simulink model "F16_2023a"  (R2025b)
settings: Solver=VariableStepAuto  StartTime=0.0  StopTime=inf  RelTol=1e-3
values from neighbouring files (symbols this model uses):
  Param = load_F16_params()    [F16AeroFM.m]    (also in runF16.m)
libraries: aerolibasang x3, aerolibfltsims x2, aerolibobsolete x1, aerolibatmos2 x1, sl3dlib x1
settings Model: Creator=sherpa  LastModifiedBy=leonardo
settings SolverCC: AlgebraicLoopSolver=TrustRegion
settings DebuggingCC: UnconnectedInputMsg=warning  UnconnectedOutputMsg=warning  UnconnectedLineMsg=warning
settings ModelReferenceCC: EnableRefExpFcnMdlSchedulingChecks=on
settings RTWCC: GPUComputeCapability=3.5  DLArmComputeVersion=19.05

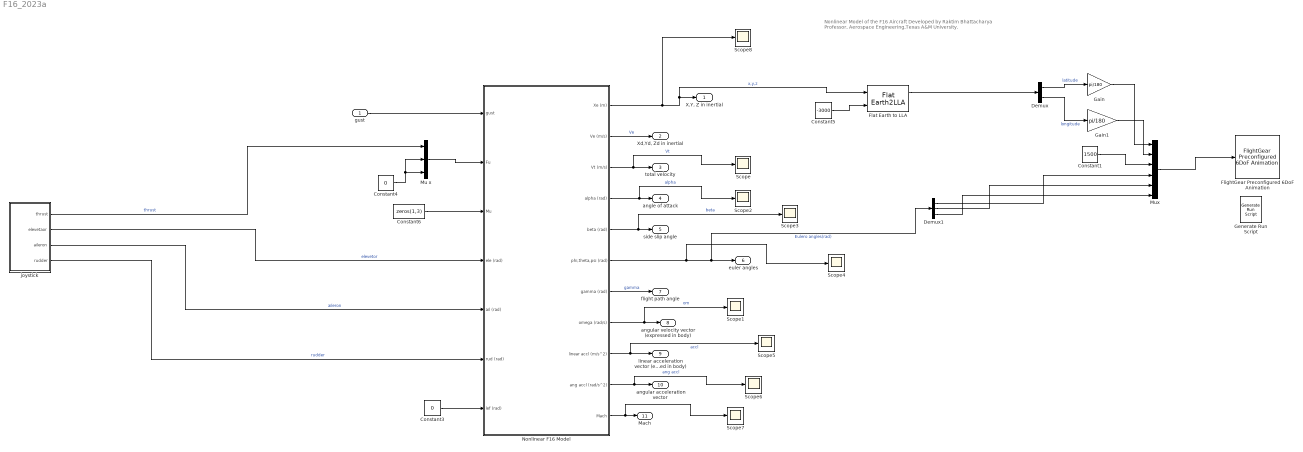
== system F16_2023a ==
  note: Nonlinear Model of the F16 Aircraft
      |
      | Developed by
      |
      | Raktim Bhattacharya
      | Professor,
      | Aerospace Engineering,Texas A&M University.
  gust : Inport
  Constant1 : Constant  Value=1500
  Constant3 : Constant  Value=0
  Constant4 : Constant  Value=0
  Constant5 : Constant  Value=-3000
  Constant6 : Constant  Value=zeros(1,3)
  Demux : Demux  Outputs=2
  Demux1 : Demux  Outputs=3
  Flat Earth to LLA : FlatEarth2LLA  LL0=[0 0]
  FlightGear Preconfigured 6DoF Animation : aerolibfltsims/FlightGear Preconfigured 6DoF Animation  xFlightGearVersion=v2019.1  DestinationIpAddress=127.0.0.1  DestinationPort=5502  SampleTime=1/30  packetVersion=24
  Gain : Gain  Gain=pi/180
  Gain1 : Gain  Gain=pi/180
  Generate Run Script : aerolibfltsims/Generate Run Script  Architecture=Linux  dataFlow=Send  GeometryModelName=c172p  AirportId=LIME  RunwayId=28  InitialAltitude=15000  InitialHeading=0  OffsetDistance=4.72  OffsetAzimuth=0  InstallScenery=off  DisableShaders=on  OriginAddress=127.0.0.1  DestinationPort=5502  OriginPort=5505  LocalAddress=127.0.0.1  OutputFileName=runfg.bat  FlightGearBaseDirectory=/usr/share/games/flightgear
  Mu x : Mux  Inputs=3
  Mux : Mux  Inputs=6
  Nonlinear F16 Model : Subsystem
  Scope{,1..8} (9 alike) : Scope
      Scope settings: ActiveDisplayYMinimum=-2227.5402486379644  ActiveDisplayYMaximum=2188.5768238395149
      Scope1 settings: ActiveDisplayYMinimum=-6.8377151322792935  ActiveDisplayYMaximum=6.6990721082944527
      Scope2 settings: ActiveDisplayYMinimum=-0.59864049768432848  ActiveDisplayYMaximum=0.52158775907311861  DataLoggingVariableName=ScopeData9
      Scope3 settings: ActiveDisplayYMinimum=-1  ActiveDisplayYMaximum=1  DataLoggingVariableName=ScopeData10
      Scope4 settings: ActiveDisplayYMinimum=-11.019979808038256  ActiveDisplayYMaximum=11.25037786436754  DataLoggingVariableName=ScopeData11
      Scope5 settings: DataLoggingVariableName=ScopeData12
      Scope6 settings: ActiveDisplayYMinimum=-1  ActiveDisplayYMaximum=1  DataLoggingVariableName=ScopeData13
      Scope7 settings: ActiveDisplayYMinimum=-1  ActiveDisplayYMaximum=1  DataLoggingVariableName=ScopeData14
      Scope8 settings: ActiveDisplayYMinimum=-126537.06226625846  ActiveDisplayYMaximum=56078.717128878794  DataLoggingVariableName=ScopeData15
  joystick : Subsystem
  "X,Y, Z in inertial" : Outport
  "Xd,Yd, Zd in inertial" : Outport  Port=2
  total velocity : Outport  Port=3
  angle of attack : Outport  Port=4
  side slip angle : Outport  Port=5
  euler angles : Outport  Port=6
  flight path angle : Outport  Port=7
  angular velocity vector (expressed in body) : Outport  Port=8
  linear acceleration vector (expressed in body) : Outport  Port=9
  angular acceleration vector : Outport  Port=10
  Mach : Outport  Port=11
  wires:
  Nonlinear F16 Model/3(Vt (m/s)) -> Scope/1, total velocity/1  "Vt"
  Nonlinear F16 Model/4(alpha (rad)) -> Scope2/1, angle of attack/1  "alpha"
  Nonlinear F16 Model/5(beta (rad)) -> Scope3/1, side slip angle/1  "beta"
  Nonlinear F16 Model/7(gamma (rad)) -> flight path angle/1  "gamma"
  Nonlinear F16 Model/8(omega (rad/s)) -> Scope1/1, angular velocity vector (expressed in body)/1  "om"
  Nonlinear F16 Model/9(linear accl (m/s^2)) -> Scope5/1, linear acceleration vector (expressed in body)/1  "accl"
  Nonlinear F16 Model/2(Ve (m/s)) -> "Xd,Yd, Zd in inertial"/1  "Ve"
  Nonlinear F16 Model/10(ang accl (rad/s^2)) -> Scope6/1, angular acceleration vector/1  "ang accl"
  Nonlinear F16 Model/11(Mach) -> Scope7/1, Mach/1
  Constant3/1 -> Nonlinear F16 Model/7(lef (rad))
  Nonlinear F16 Model/6(phi,theta,psi (rad)) -> Scope4/1, Demux1/1, euler angles/1  "Eulero angles(rad)"
  Nonlinear F16 Model/1(Xe (m)) -> Scope8/1, Flat Earth to LLA/1, "X,Y, Z in inertial"/1  "x,y,z"
  Constant4/1 -> Mu x/2, Mu x/3
  Mu x/1 -> Nonlinear F16 Model/2(Fu)
  Flat Earth to LLA/1 -> Demux/1
  Constant5/1 -> Flat Earth to LLA/2
  Constant6/1 -> Nonlinear F16 Model/3(Mu)
  Demux/1 -> Gain/1  "latitude"
  Demux/2 -> Gain1/1  "longitude"
  Mux/1 -> FlightGear Preconfigured 6DoF Animation/1
  Demux1/1 -> Mux/4
  Demux1/2 -> Mux/5
  Constant1/1 -> Mux/3
  gust/1 -> Nonlinear F16 Model/1(gust)
  joystick/1(thrust) -> Mu x/1  "thrust"
  joystick/2(elevetaor) -> Nonlinear F16 Model/4(ele (rad))  "elevetor"
  joystick/3(aileron) -> Nonlinear F16 Model/5(ail (rad))  "aileron"
  joystick/4(rudder) -> Nonlinear F16 Model/6(rud (rad))  "rudder"
  Demux1/3 -> Mux/6
  Gain/1 -> Mux/1
  Gain1/1 -> Mux/2

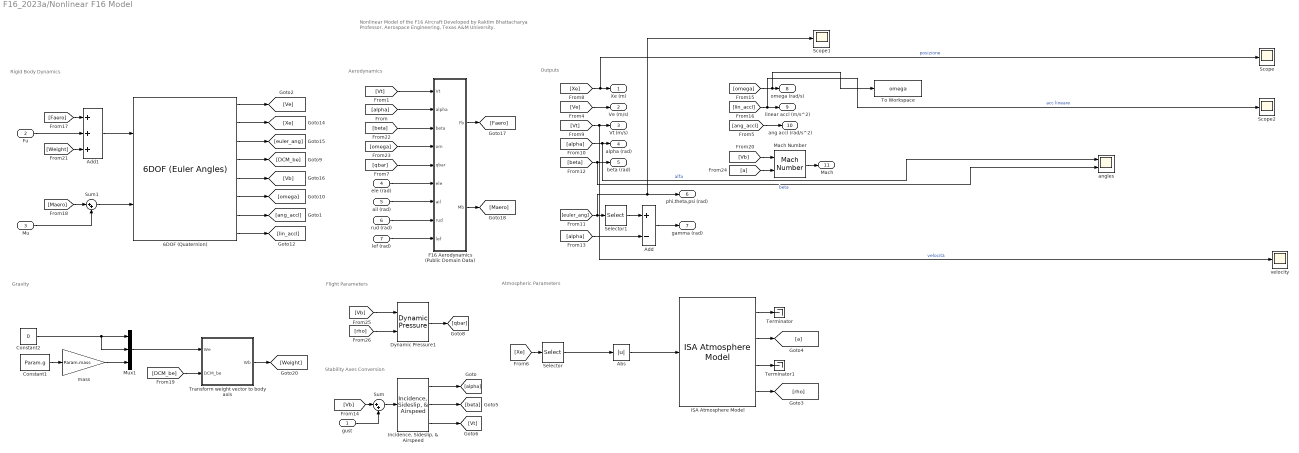
== system F16_2023a/Nonlinear F16 Model ==
  note: Gravity
  note: Nonlinear Model of the F16 Aircraft
      |
      | Developed by Raktim Bhattacharya
      | Professor, Aerospace Engineering,
      | Texas A&M University.
  note: Aerodynamics
  note: Outputs
  note: Rigid Body Dynamics
  note: Stability Axes Conversion
  note: Atmospheric Parameters
  note: Flight Parameters
  gust : Inport  PortDimensions=3
  Fu : Inport  Port=2  PortDimensions=3
  Mu : Inport  Port=3  PortDimensions=3
  ele (rad) : Inport  Port=4
  ail (rad) : Inport  Port=5
  rud (rad) : Inport  Port=6
  lef (rad) : Inport  Port=7
  6DOF (Quaternion) : aerolibobsolete/6DOF (Euler Angles)  units=Metric (MKS)  mtype=Fixed  rep=Euler Angles  xme_0=IC.inertial_position  Vm_0=IC.body_velocity  eul_0=IC.euler_angles  pm_0=IC.omega  mass_0=Param.mass  mass_e=0.5  mass_f=2.0  inertia=Param.moi  inertia_e=eye(3)  inertia_f=2*eye(3)  k_quat=1.0  vre_flag=on  abi_flag=off  aMode=0  xme_statename={'Xe', 'Ye', 'Ze'}  Vm_statename={'U', 'v', 'w'}  eul_statename=''  quat_statename={'qr', 'qi', 'qj', 'qk'}  pm_statename={'p', 'q', 'r'}  mass_statename=''
  Abs : Abs  SaturateOnIntegerOverflow=off
  Add : Sum  Inputs=+-
  Add1 : Sum  Inputs=+++
  Constant1 : Constant  Value=Param.g
  Constant2 : Constant  Value=0
  Dynamic Pressure1 : aerolibasang/Dynamic Pressure
  F16 Aerodynamics (Public Domain Data) : Subsystem
  ISA Atmosphere Model : aerolibatmos2/ISA Atmosphere Model  useExtended=off  action=None  custom=off  viscosityOut=off  g=9.80665  gamma=1.4  R=287.0531  L=0.0065  h_trop=11000  h_strat=20000  rho0=1.225  P0=101325  T0=288.15  h0=0  S=110.4  Tref=273.15  muref=1.716e-5
  "Incidence, Sideslip, & Airspeed" : aerolibasang/Incidence, Sideslip, & Airspeed
  Mach Number : aerolibasang/Mach Number
  Mux1 : Mux  Inputs=3
  Scope : Scope
      settings: ActiveDisplayYMinimum=-9160.141053235342  ActiveDisplayYMaximum=5347.118129523169  DataLoggingVariableName=ScopeData2
  Scope1 : Scope
      settings: ActiveDisplayYMinimum=-2.5924276815871528  ActiveDisplayYMaximum=1.1099100940481796  DataLoggingVariableName=ScopeData3
  Scope2 : Scope
      settings: ActiveDisplayYMinimum=-38.16136847895087  ActiveDisplayYMaximum=61.768795303374354  DataLoggingVariableName=ScopeData5
  Selector : Selector  InputPortWidth=3  IndexOptions=Index vector (dialog)  Indices=3  OutputSizes=1
  Selector1 : Selector  InputPortWidth=3  IndexOptions=Index vector (dialog)  Indices=2  OutputSizes=1
  Sum : Sum  Inputs=|++
  Sum1 : Sum  Inputs=|++
  Terminator : Terminator
  Terminator1 : Terminator
  To Workspace : ToWorkspace  VariableName=omega  SaveFormat=Timeseries  SampleTime=-1
  Transform weight vector to body axis : MATLAB Function  TreatAsAtomicUnit=on
  angles : Scope  NumInputPorts=2
      settings: ActiveDisplayYMinimum=-0.37545003667394233  ActiveDisplayYMaximum=0.11642688367935129  DataLoggingVariableName=ScopeData4
  mass : Gain  Gain=Param.mass
  velocity : Scope
      settings: ActiveDisplayYMinimum=59.795753806398508  ActiveDisplayYMaximum=111.44827585460112  DataLoggingVariableName=ScopeData6
  Xe (m) : Outport
  Ve (m/s) : Outport  Port=2
  Vt (m/s) : Outport  Port=3
  alpha (rad) : Outport  Port=4
  beta (rad) : Outport  Port=5
  phi,theta,psi (rad) : Outport  Port=6
  gamma (rad) : Outport  Port=7
  omega (rad/s) : Outport  Port=8
  linear accl (m/s^2) : Outport  Port=9
  ang accl (rad/s^2) : Outport  Port=10
  Mach : Outport  Port=11
  wires:
  [Xe] -> Selector/1
  [beta] -> angles/2, beta (rad)/1  "beta"
  "Incidence, Sideslip, & Airspeed"/3 -> [Vt]
  ISA Atmosphere Model/3 -> Terminator1/1
  ISA Atmosphere Model/1 -> Terminator/1
  ISA Atmosphere Model/4 -> [rho]
  [lin_accl] -> Scope2/1, linear accl (m/s^2)/1  "acc lineare"
  [alpha] -> angles/1, alpha (rad)/1  "alfa"
  ISA Atmosphere Model/2 -> [a]
  Add/1 -> gamma (rad)/1
  [Vt] -> velocity/1, Vt (m/s)/1  "velocità"
  "Incidence, Sideslip, & Airspeed"/2 -> [beta]
  Selector1/1 -> Add/1
  "Incidence, Sideslip, & Airspeed"/1 -> [alpha]
  Selector/1 -> Abs/1
  [alpha] -> Add/2
  [euler_ang] -> Scope1/1, phi,theta,psi (rad)/1, Selector1/1
  [omega] -> To Workspace/1, omega (rad/s)/1
  [Xe] -> Scope/1, Xe (m)/1  "posizione"
  Constant1/1 -> mass/1
  mass/1 -> Mux1/3
  Mux1/1 -> Transform weight vector to body axis/1(We)
  Transform weight vector to body axis/1(Wb) -> [Weight]
  [DCM_be] -> Transform weight vector to body axis/2(DCM_be)
  Constant2/1 -> Mux1/2, Mux1/1
  [Faero] -> Add1/1
  Fu/1 -> Add1/2
  [Weight] -> Add1/3
  Add1/1 -> 6DOF (Quaternion)/1
  [Vb] -> Sum/1
  Sum/1 -> "Incidence, Sideslip, & Airspeed"/1
  gust/1 -> Sum/2
  [Maero] -> Sum1/1
  Mu/1 -> Sum1/2
  6DOF (Quaternion)/1 -> [Ve]
  6DOF (Quaternion)/2 -> [Xe]
  6DOF (Quaternion)/3 -> [euler_ang]
  6DOF (Quaternion)/4 -> [DCM_be]
  6DOF (Quaternion)/5 -> [Vb]
  6DOF (Quaternion)/6 -> [omega]
  6DOF (Quaternion)/7 -> [ang_accl]
  6DOF (Quaternion)/8 -> [lin_accl]
  [Ve] -> Ve (m/s)/1
  [ang_accl] -> ang accl (rad/s^2)/1
  [Vb] -> Mach Number/1
  [a] -> Mach Number/2
  Mach Number/1 -> Mach/1
  F16 Aerodynamics (Public Domain Data)/1(Fb) -> [Faero]
  Sum1/1 -> 6DOF (Quaternion)/2
  F16 Aerodynamics (Public Domain Data)/2(Mb) -> [Maero]
  [Vt] -> F16 Aerodynamics (Public Domain Data)/1(Vt)
  [alpha] -> F16 Aerodynamics (Public Domain Data)/2(alpha)
  [beta] -> F16 Aerodynamics (Public Domain Data)/3(beta)
  [omega] -> F16 Aerodynamics (Public Domain Data)/4(om)
  [qbar] -> F16 Aerodynamics (Public Domain Data)/5(qbar)
  ele (rad)/1 -> F16 Aerodynamics (Public Domain Data)/6(ele)
  ail (rad)/1 -> F16 Aerodynamics (Public Domain Data)/7(ail)
  rud (rad)/1 -> F16 Aerodynamics (Public Domain Data)/8(rud)
  lef (rad)/1 -> F16 Aerodynamics (Public Domain Data)/9(lef)
  Abs/1 -> ISA Atmosphere Model/1
  Dynamic Pressure1/1 -> [qbar]
  [Vb] -> Dynamic Pressure1/1
  [rho] -> Dynamic Pressure1/2

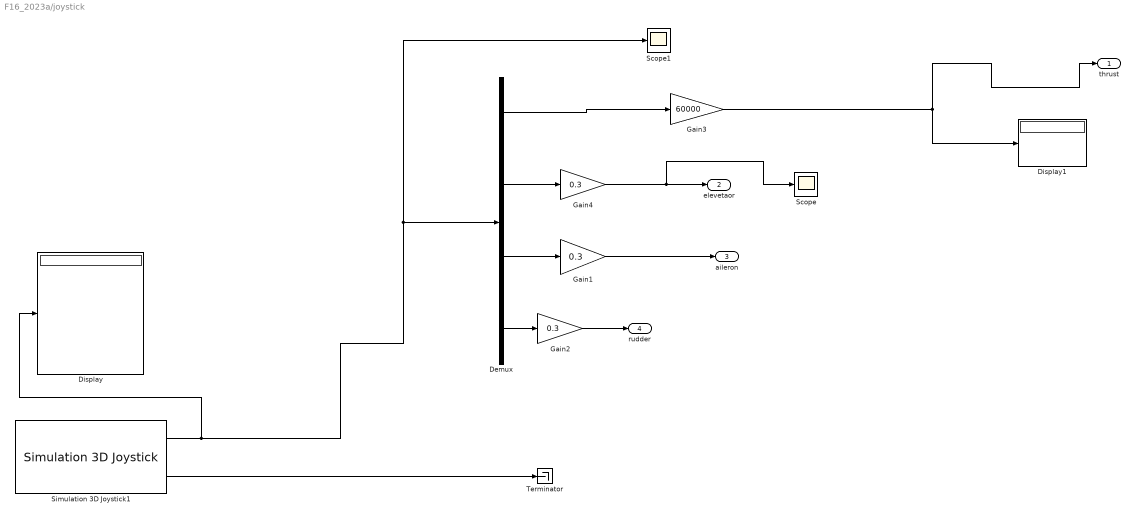
== system F16_2023a/joystick ==
  Demux : Demux
  Display : Display
  Display1 : Display
  Gain1 : Gain  Gain=0.3
  Gain2 : Gain  Gain=0.3
  Gain3 : Gain  Gain=60000
  Gain4 : Gain  Gain=0.3
  Scope : Scope
      settings: ActiveDisplayYMinimum=-0.18749999999999997  ActiveDisplayYMaximum=0.18749999999999997  DataLoggingVariableName=ScopeData7
  Scope1 : Scope
      settings: ActiveDisplayYMinimum=-12.345890787364121  ActiveDisplayYMaximum=10.806609212635932  DataLoggingVariableName=ScopeData8
  Simulation 3D Joystick1 : sl3dlib/Simulation 3D/Hardware Interface/Simulation 3D Joystick  joyid=1  adjustports=on  forcefeed=off
  Terminator : Terminator
  thrust : Outport
  elevetaor : Outport  Port=2
  aileron : Outport  Port=3
  rudder : Outport  Port=4
  wires:
  Gain4/1 -> Scope/1, elevetaor/1
  Gain1/1 -> aileron/1
  Gain2/1 -> rudder/1
  Simulation 3D Joystick1/1 -> Scope1/1, Demux/1, Display/1
  Simulation 3D Joystick1/2 -> Terminator/1
  Gain3/1 -> thrust/1, Display1/1
  Demux/4 -> Gain2/1
  Demux/1 -> Gain3/1
  Demux/2 -> Gain4/1
  Demux/3 -> Gain1/1

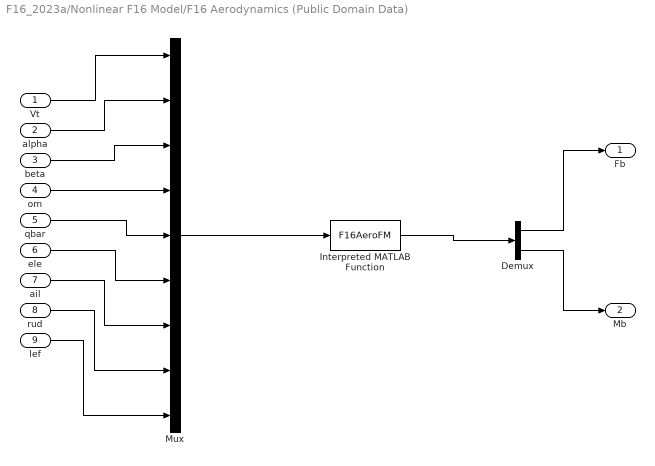
== system F16_2023a/Nonlinear F16 Model/F16 Aerodynamics (Public Domain Data) ==
  Vt : Inport
  alpha : Inport  Port=2
  beta : Inport  Port=3
  om : Inport  Port=4
  qbar : Inport  Port=5
  ele : Inport  Port=6
  ail : Inport  Port=7
  rud : Inport  Port=8
  lef : Inport  Port=9
  Demux : Demux  Outputs=2
  Interpreted MATLAB Function : MATLABFcn  MATLABFcn=F16AeroFM  OutputDimensions=6
  Mux : Mux  Inputs=9
  Fb : Outport  PortDimensions=3
  Mb : Outport  Port=2  PortDimensions=3
  wires:
  om/1 -> Mux/4
  beta/1 -> Mux/3
  qbar/1 -> Mux/5
  alpha/1 -> Mux/2
  ele/1 -> Mux/6
  Vt/1 -> Mux/1
  ail/1 -> Mux/7
  rud/1 -> Mux/8
  lef/1 -> Mux/9
  Mux/1 -> Interpreted MATLAB Function/1
  Demux/1 -> Fb/1
  Demux/2 -> Mb/1
  Interpreted MATLAB Function/1 -> Demux/1

== matlab function F16_2023a/Nonlinear F16 Model/Transform weight vector to body axis ==
  data: We input; Wb output; DCM_be input
function Wb = fcn(We,DCM_be)
Wb = DCM_be*We; % Weight in body coordinate system. DCM_be is correct, no need for transpose. They must have fixed it in this version.
